simulink model "fangzhen"  (R2020b)
settings: Solver=VariableStepAuto  StartTime=0.0  StopTime=10.0  RelTol=1e-3
settings Model: Creator=86152  LastModifiedBy=86152

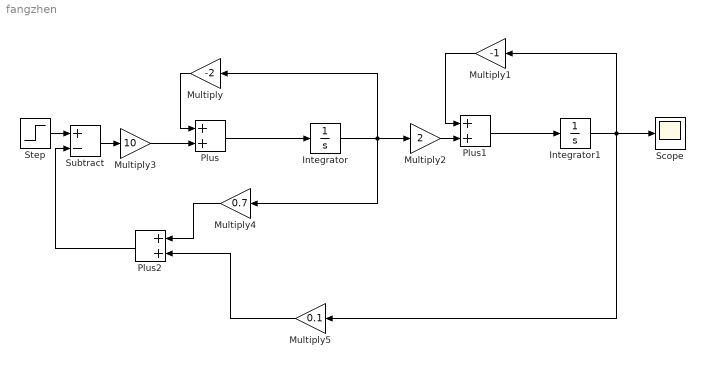
== system fangzhen ==
  Integrator : Integrator
  Integrator1 : Integrator
  Multiply : Gain  Gain=-2
  Multiply1 : Gain  Gain=-1
  Multiply2 : Gain  Gain=2
  Multiply3 : Gain  Gain=10
  Multiply4 : Gain  Gain=0.7
  Multiply5 : Gain  Gain=0.1
  Plus : Sum
  Plus1 : Sum
  Plus2 : Sum
  Scope : Scope
  Step : Step  Time=0  SampleTime=0
  Subtract : Sum  Inputs=+-
  wires:
  Plus/1 -> Integrator/1
  Multiply/1 -> Plus/1
  Integrator/1 -> Multiply4/1, Multiply2/1, Multiply/1
  Plus1/1 -> Integrator1/1
  Multiply2/1 -> Plus1/2
  Multiply1/1 -> Plus1/1
  Multiply3/1 -> Plus/2
  Step/1 -> Subtract/1
  Subtract/1 -> Multiply3/1
  Integrator1/1 -> Multiply5/1, Multiply1/1, Scope/1
  Plus2/1 -> Subtract/2
  Multiply4/1 -> Plus2/1
  Multiply5/1 -> Plus2/2
